simulink model "Model_OnlyDark_17_10_11_hperrorsign_nocs_nocorrel"  (R2015a)
settings: Solver=FixedStepDiscrete  StartTime=0.0  StopTime=5  FixedStep=0.001  RelTol=1e-3
InitFcn:
  | %Ts=parameter.Ts;
  |    %Sampling Time, 50 times slower than original model
model workspace (MAT data in the model file):
  padsize = 8
  x1 = 14
undefined symbols (not defined in the file): alpha_downslope_off, alpha_downslope_on, alpha_upslope_off, alpha_upslope_on
settings Model: tstep=0.1  TimeStep=0.1  CovSFcnEnable=off  Creator=a1174239  LastModifiedBy=John
settings SolverCC: AlgebraicLoopSolver=LineSearch
settings DataIOCC: MaxDataPoints=1
settings OptimizationCC: ExpressionDepthLimit=2147483647  EfficientMapNaN2IntZero=off
settings DebuggingCC: UnderspecifiedInitializationDetection=Classic  MergeDetectMultiDrivingBlocksExec=none  SolverPrmCheckMsg=warning  MultiTaskDSMMsg=warning  MultiTaskCondExecSysMsg=none  ParameterPrecisionLossMsg=none  StateNameClashWarn=warning
settings HardwareCC: TargetLongLongMode=on  TargetIntDivRoundTo=Zero  TargetEndianess=LittleEndian  TargetHWDeviceType=MATLAB Host  ProdEqTarget=off
settings CodeAppCC: MaxIdLength=128
settings GRTTargetCC: CombineOutputUpdateFcns=off  GRTInterface=on

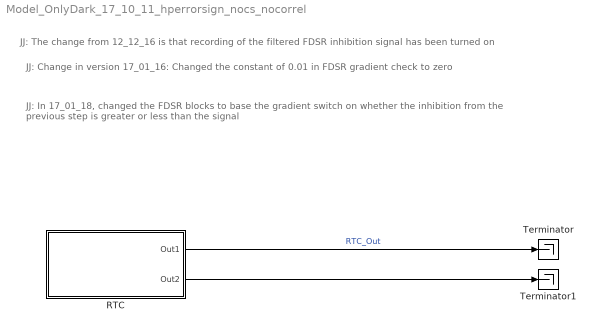
== system Model_OnlyDark_17_10_11_hperrorsign_nocs_nocorrel ==
  note: JJ: In 17_01_18, changed the FDSR blocks to base the gradient switch on whether the inhibition from the previous step is greater or less than the signal
  note: JJ: Change in version 17_01_16: Changed the constant of 0.01 in FDSR gradient check to zero
  note: JJ: The change from 12_12_16 is that recording of the filtered FDSR inhibition signal has been turned on
  RTC : Subsystem
  Terminator : Terminator
  Terminator1 : Terminator
  wires:
  RTC/1(Out1) -> Terminator/1  "RTC_Out"
  RTC/2(Out2) -> Terminator1/1

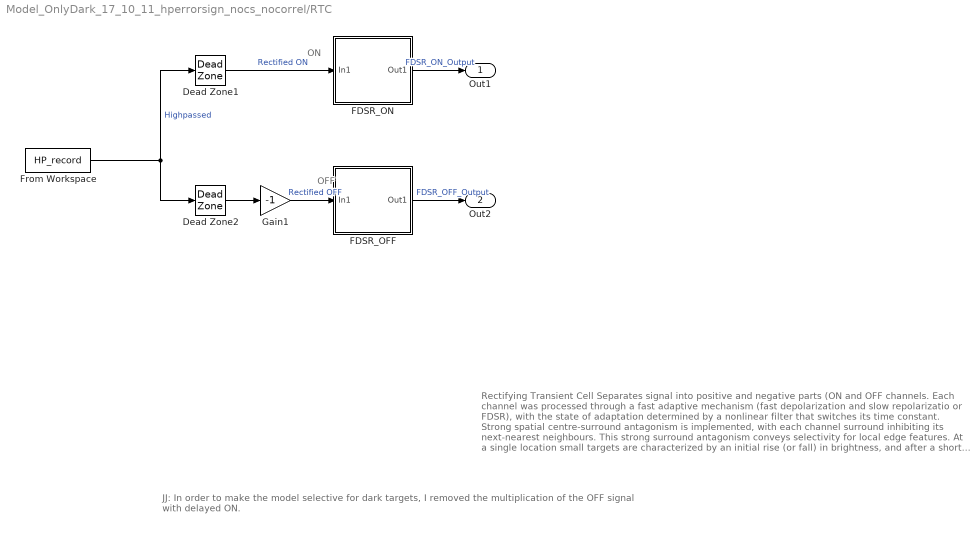
== system Model_OnlyDark_17_10_11_hperrorsign_nocs_nocorrel/RTC ==
  note: JJ: In order to make the model selective for dark targets, I removed the multiplication of the OFF signal with delayed ON.
  note: ON
  note: OFF
  note: Rectifying Transient Cell Separates signal into positive and negative parts (ON and OFF channels. Each channel was processed through a fast adaptive mechanism (fast depolarization and slow repolarizatio or FDSR),
      | with the state of adaptation determined by a nonlinear filter that switches its time constant. Strong spatial centre-surround antagonism is implemented, with each channel surround inhibiting its next-nearest neighbours.
      | This strong surround antagonism conveys selectivity for local edge features. At a single location small targets are characterized by an initial rise (or fall) in brightness, and after a short delay are followed by a corresponding
      | fall (or rise), irrespective of the direction of travel. Sensitivity to targets independent of their polarity was provided by multiplying each contrast channel (ON or OFF) with a delayed version of the opposite polarity
      | (via a low-pass filter,) and then summing the outputs.
  Dead Zone1 : DeadZone  LowerValue=-inf  UpperValue=0  SaturateOnIntegerOverflow=on
  Dead Zone2 : DeadZone  LowerValue=0  UpperValue=inf  SaturateOnIntegerOverflow=on
  FDSR_OFF : Subsystem
  FDSR_ON : Subsystem
  From Workspace : FromWorkspace  VariableName=HP_record  SampleTime=0.001  Interpolate=off  OutputAfterFinalValue=Setting to zero
  Gain1 : Gain  Gain=-1
  Out1 : Outport
  Out2 : Outport  Port=2
  wires:
  Gain1/1 -> FDSR_OFF/1(In1)  "Rectified OFF"
  Dead Zone1/1 -> FDSR_ON/1(In1)  "Rectified ON"
  Dead Zone2/1 -> Gain1/1
  From Workspace/1 -> Dead Zone2/1, Dead Zone1/1  "Highpassed"
  FDSR_OFF/1(Out1) -> Out2/1  "FDSR_OFF_Output"
  FDSR_ON/1(Out1) -> Out1/1  "FDSR_ON_Output"

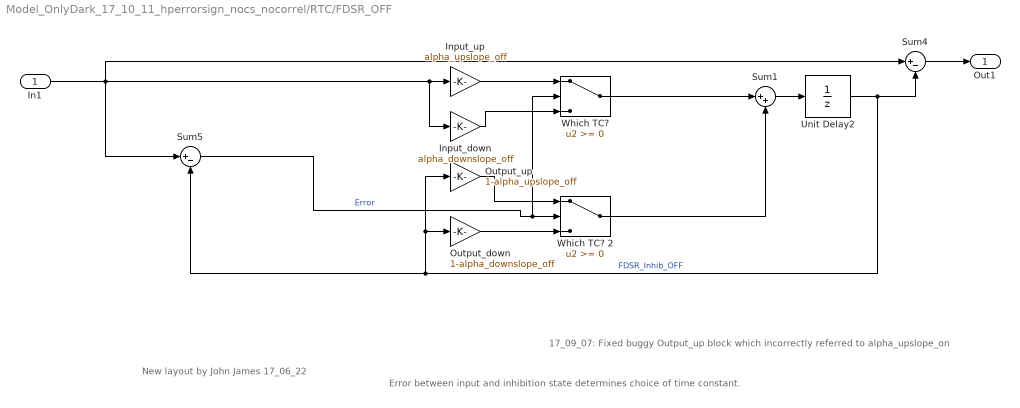
== system Model_OnlyDark_17_10_11_hperrorsign_nocs_nocorrel/RTC/FDSR_OFF ==
  note: 17_09_07: Fixed buggy Output_up block which incorrectly referred to alpha_upslope_on
  note: Error between input and inhibition state determines choice of time constant.
  note: New layout by John James 17_06_22
  In1 : Inport
  Input_down : Gain  Gain=alpha_downslope_off
  Input_up : Gain  Gain=alpha_upslope_off
  Output_down : Gain  Gain=1-alpha_downslope_off
  Output_up : Gain  Gain=1-alpha_upslope_off
  Sum1 : Sum  Inputs=|++
  Sum4 : Sum  Inputs=|+-
  Sum5 : Sum  Inputs=|+-
  Unit Delay2 : UnitDelay  InitialCondition=[2.092691e-02 6.806062e-03 1.030208e-02 1.714690e-02 1.904537e-02 2.139582e-02 3.714136e-02 ;1.756770e-02 8.333369e-03 1.093624e-02 1.157973e-02 2.179743e-02 2.285020e-02 4.216066e-02 ;1.626654e-02 2.800405e-02 4.677293e-02 1.656982e-02 2.217366e-02 2.716260e-02 4.415135e-02 ;5.502986e-02 8.236043e-02 6.068115e-02 2.302062e-02 1.836370e-02 3.141778e-02 2.534562e-02 ;3.135326e-02 2.317981e-02 3.244115e-02 8.679342e-03 9.377349e-03 9.338796e-03 1.375442e-02 ;1.668327e-02 1.177946e-02 2.244038e-02 2.842079e-02 1.103765e-02 3.728219e-03 5.666695e-03 ;1.030520e-02 7.595676e-03 6.415971e-03 6.775899e-03 1.118897e-02 3.894019e-03 2.353740e-03]  SampleTime=-1
  Which TC? : Switch
  Which TC? 2 : Switch
  Out1 : Outport
  wires:
  In1/1 -> Input_down/1, Input_up/1, Sum5/1, Sum4/1
  Input_up/1 -> Which TC?/1
  Input_down/1 -> Which TC?/3
  Output_up/1 -> Which TC? 2/1
  Output_down/1 -> Which TC? 2/3
  Which TC?/1 -> Sum1/1
  Which TC? 2/1 -> Sum1/2
  Sum4/1 -> Out1/1
  Sum1/1 -> Unit Delay2/1
  Unit Delay2/1 -> Sum5/2, Output_up/1, Output_down/1, Sum4/2  "FDSR_Inhib_OFF"
  Sum5/1 -> Which TC?/2, Which TC? 2/2  "Error"

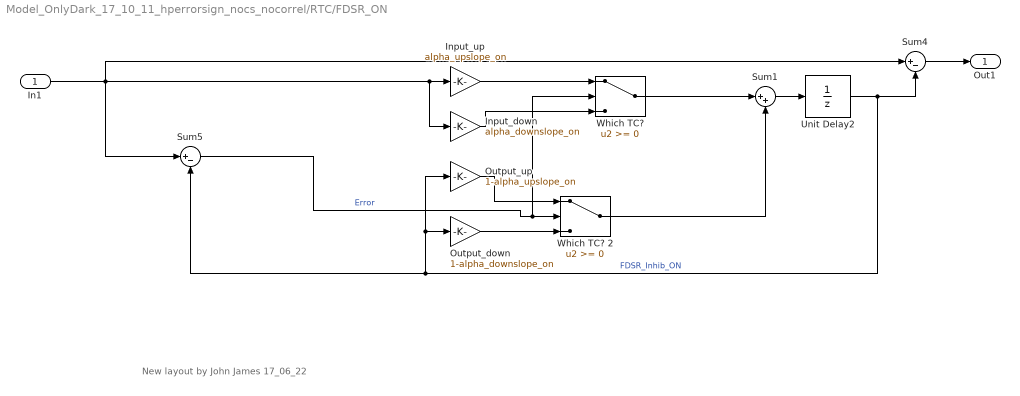
== system Model_OnlyDark_17_10_11_hperrorsign_nocs_nocorrel/RTC/FDSR_ON ==
  note: New layout by John James 17_06_22
  In1 : Inport
  Input_down : Gain  Gain=alpha_downslope_on
  Input_up : Gain  Gain=alpha_upslope_on
  Output_down : Gain  Gain=1-alpha_downslope_on
  Output_up : Gain  Gain=1-alpha_upslope_on
  Sum1 : Sum  Inputs=|++
  Sum4 : Sum  Inputs=|+-
  Sum5 : Sum  Inputs=|+-
  Unit Delay2 : UnitDelay  SampleTime=-1
  Which TC? : Switch
  Which TC? 2 : Switch
  Out1 : Outport
  wires:
  In1/1 -> Input_down/1, Input_up/1, Sum5/1, Sum4/1
  Input_up/1 -> Which TC?/1
  Input_down/1 -> Which TC?/3
  Output_up/1 -> Which TC? 2/1
  Output_down/1 -> Which TC? 2/3
  Which TC?/1 -> Sum1/1
  Which TC? 2/1 -> Sum1/2
  Sum4/1 -> Out1/1
  Sum1/1 -> Unit Delay2/1
  Unit Delay2/1 -> Sum5/2, Output_up/1, Output_down/1, Sum4/2  "FDSR_Inhib_ON"
  Sum5/1 -> Which TC?/2, Which TC? 2/2  "Error"
